simulink model "hx_model_alsop_20stages"  (R2017b)
settings: Solver=FixedStepAuto  StartTime=0.0  StopTime=Tsim  FixedStep=ST  RelTol=1e-3
values from neighbouring files (symbols this model uses):
  a1 = N_stages/(3600*Mc)    (= 0.000138888888889)    [main_open_loop_step_responses.m]    (also in main_pida_vs_pid_Fp_dist.m; main_pida_vs_pid_Tci_dist.m; main_pida_vs_pid_Tpi_dist.m; main_pida_vs_pid_sp.m)
  a2 = (U*A)/(3600*Mc*Cpc)    (= 0.010660331384)    [main_open_loop_step_responses.m]    (also in main_pida_vs_pid_Fp_dist.m; main_pida_vs_pid_Tci_dist.m; main_pida_vs_pid_Tpi_dist.m; main_pida_vs_pid_sp.m)
  a3 = N_stages/(3600*Mp)    (= 0.00037037037037)    [main_open_loop_step_responses.m]    (also in main_pida_vs_pid_Fp_dist.m; main_pida_vs_pid_Tci_dist.m; main_pida_vs_pid_Tpi_dist.m; main_pida_vs_pid_sp.m)
  a4 = (U*A)/(3600*Mp*Cpp)    (= 0.0341130604288)    [main_open_loop_step_responses.m]    (also in main_pida_vs_pid_Fp_dist.m; main_pida_vs_pid_Tci_dist.m; main_pida_vs_pid_Tpi_dist.m; main_pida_vs_pid_sp.m)
  Fc = 2500/7936.64    (= 0.314994758487)    [main_open_loop_step_responses.m]    (also in main_pida_vs_pid_Fp_dist.m; main_pida_vs_pid_Tci_dist.m; main_pida_vs_pid_Tpi_dist.m; main_pida_vs_pid_sp.m)
  Fp = 1500/7936.64    (= 0.188996855092)    [main_open_loop_step_responses.m]    (also in main_pida_vs_pid_Fp_dist.m; main_pida_vs_pid_Tci_dist.m; main_pida_vs_pid_Tpi_dist.m; main_pida_vs_pid_sp.m)
  step_Fc = -0.15    [main_open_loop_step_responses.m]    (also in main_tuning_pid.m = -0.05; main_tuning_pida.m = -0.05)
  step_time = 0    [main_open_loop_step_responses.m]    (also in main_pida_vs_pid_Fp_dist.m; main_pida_vs_pid_Tci_dist.m; main_pida_vs_pid_Tpi_dist.m; main_pida_vs_pid_sp.m)
  Tci = 294.26    [main_open_loop_step_responses.m]    (also in main_pida_vs_pid_Fp_dist.m; main_pida_vs_pid_Tci_dist.m; main_pida_vs_pid_Tpi_dist.m; main_pida_vs_pid_sp.m)
  Tco_init1 = Tco_init1.Data(end)    [main_open_loop_step_responses.m]    (also in main_pida_vs_pid_Fp_dist.m; main_pida_vs_pid_Tci_dist.m; main_pida_vs_pid_Tpi_dist.m; main_pida_vs_pid_sp.m)
  Tco_init10 = Tco_init10.Data(end)    [main_open_loop_step_responses.m]    (also in main_pida_vs_pid_Fp_dist.m; main_pida_vs_pid_Tci_dist.m; main_pida_vs_pid_Tpi_dist.m; main_pida_vs_pid_sp.m)
  Tco_init11 = Tco_init11.Data(end)    [main_open_loop_step_responses.m]    (also in main_pida_vs_pid_Fp_dist.m; main_pida_vs_pid_Tci_dist.m; main_pida_vs_pid_Tpi_dist.m; main_pida_vs_pid_sp.m)
  Tco_init12 = Tco_init12.Data(end)    [main_open_loop_step_responses.m]    (also in main_pida_vs_pid_Fp_dist.m; main_pida_vs_pid_Tci_dist.m; main_pida_vs_pid_Tpi_dist.m; main_pida_vs_pid_sp.m)
  Tco_init13 = Tco_init13.Data(end)    [main_open_loop_step_responses.m]    (also in main_pida_vs_pid_Fp_dist.m; main_pida_vs_pid_Tci_dist.m; main_pida_vs_pid_Tpi_dist.m; main_pida_vs_pid_sp.m)
  Tco_init14 = Tco_init14.Data(end)    [main_open_loop_step_responses.m]    (also in main_pida_vs_pid_Fp_dist.m; main_pida_vs_pid_Tci_dist.m; main_pida_vs_pid_Tpi_dist.m; main_pida_vs_pid_sp.m)
  Tco_init15 = Tco_init15.Data(end)    [main_open_loop_step_responses.m]    (also in main_pida_vs_pid_Fp_dist.m; main_pida_vs_pid_Tci_dist.m; main_pida_vs_pid_Tpi_dist.m; main_pida_vs_pid_sp.m)
  Tco_init16 = Tco_init16.Data(end)    [main_open_loop_step_responses.m]    (also in main_pida_vs_pid_Fp_dist.m; main_pida_vs_pid_Tci_dist.m; main_pida_vs_pid_Tpi_dist.m; main_pida_vs_pid_sp.m)
  Tco_init17 = Tco_init17.Data(end)    [main_open_loop_step_responses.m]    (also in main_pida_vs_pid_Fp_dist.m; main_pida_vs_pid_Tci_dist.m; main_pida_vs_pid_Tpi_dist.m; main_pida_vs_pid_sp.m)
  Tco_init18 = Tco_init18.Data(end)    [main_open_loop_step_responses.m]    (also in main_pida_vs_pid_Fp_dist.m; main_pida_vs_pid_Tci_dist.m; main_pida_vs_pid_Tpi_dist.m; main_pida_vs_pid_sp.m)
  Tco_init19 = Tco_init19.Data(end)    [main_open_loop_step_responses.m]    (also in main_pida_vs_pid_Fp_dist.m; main_pida_vs_pid_Tci_dist.m; main_pida_vs_pid_Tpi_dist.m; main_pida_vs_pid_sp.m)
  Tco_init2 = Tco_init2.Data(end)    [main_open_loop_step_responses.m]    (also in main_pida_vs_pid_Fp_dist.m; main_pida_vs_pid_Tci_dist.m; main_pida_vs_pid_Tpi_dist.m; main_pida_vs_pid_sp.m)
  Tco_init20 = Tco_init20.Data(end)    [main_open_loop_step_responses.m]    (also in main_pida_vs_pid_Fp_dist.m; main_pida_vs_pid_Tci_dist.m; main_pida_vs_pid_Tpi_dist.m; main_pida_vs_pid_sp.m)
  Tco_init3 = Tco_init3.Data(end)    [main_open_loop_step_responses.m]    (also in main_pida_vs_pid_Fp_dist.m; main_pida_vs_pid_Tci_dist.m; main_pida_vs_pid_Tpi_dist.m; main_pida_vs_pid_sp.m)
  Tco_init4 = Tco_init4.Data(end)    [main_open_loop_step_responses.m]    (also in main_pida_vs_pid_Fp_dist.m; main_pida_vs_pid_Tci_dist.m; main_pida_vs_pid_Tpi_dist.m; main_pida_vs_pid_sp.m)
  Tco_init5 = Tco_init5.Data(end)    [main_open_loop_step_responses.m]    (also in main_pida_vs_pid_Fp_dist.m; main_pida_vs_pid_Tci_dist.m; main_pida_vs_pid_Tpi_dist.m; main_pida_vs_pid_sp.m)
  Tco_init6 = Tco_init6.Data(end)    [main_open_loop_step_responses.m]    (also in main_pida_vs_pid_Fp_dist.m; main_pida_vs_pid_Tci_dist.m; main_pida_vs_pid_Tpi_dist.m; main_pida_vs_pid_sp.m)
  Tco_init7 = Tco_init7.Data(end)    [main_open_loop_step_responses.m]    (also in main_pida_vs_pid_Fp_dist.m; main_pida_vs_pid_Tci_dist.m; main_pida_vs_pid_Tpi_dist.m; main_pida_vs_pid_sp.m)
  Tco_init8 = Tco_init8.Data(end)    [main_open_loop_step_responses.m]    (also in main_pida_vs_pid_Fp_dist.m; main_pida_vs_pid_Tci_dist.m; main_pida_vs_pid_Tpi_dist.m; main_pida_vs_pid_sp.m)
  Tco_init9 = Tco_init9.Data(end)    [main_open_loop_step_responses.m]    (also in main_pida_vs_pid_Fp_dist.m; main_pida_vs_pid_Tci_dist.m; main_pida_vs_pid_Tpi_dist.m; main_pida_vs_pid_sp.m)
  Tpi = 366.48    [main_open_loop_step_responses.m]    (also in main_pida_vs_pid_Fp_dist.m; main_pida_vs_pid_Tci_dist.m; main_pida_vs_pid_Tpi_dist.m; main_pida_vs_pid_sp.m)
  Tpo_init1 = Tpo_init1.Data(end)    [main_open_loop_step_responses.m]    (also in main_pida_vs_pid_Fp_dist.m; main_pida_vs_pid_Tci_dist.m; main_pida_vs_pid_Tpi_dist.m; main_pida_vs_pid_sp.m)
  Tpo_init10 = Tpo_init10.Data(end)    [main_open_loop_step_responses.m]    (also in main_pida_vs_pid_Fp_dist.m; main_pida_vs_pid_Tci_dist.m; main_pida_vs_pid_Tpi_dist.m; main_pida_vs_pid_sp.m)
  Tpo_init11 = Tpo_init11.Data(end)    [main_open_loop_step_responses.m]    (also in main_pida_vs_pid_Fp_dist.m; main_pida_vs_pid_Tci_dist.m; main_pida_vs_pid_Tpi_dist.m; main_pida_vs_pid_sp.m)
  Tpo_init12 = Tpo_init12.Data(end)    [main_open_loop_step_responses.m]    (also in main_pida_vs_pid_Fp_dist.m; main_pida_vs_pid_Tci_dist.m; main_pida_vs_pid_Tpi_dist.m; main_pida_vs_pid_sp.m)
  Tpo_init13 = Tpo_init13.Data(end)    [main_open_loop_step_responses.m]    (also in main_pida_vs_pid_Fp_dist.m; main_pida_vs_pid_Tci_dist.m; main_pida_vs_pid_Tpi_dist.m; main_pida_vs_pid_sp.m)
  Tpo_init14 = Tpo_init14.Data(end)    [main_open_loop_step_responses.m]    (also in main_pida_vs_pid_Fp_dist.m; main_pida_vs_pid_Tci_dist.m; main_pida_vs_pid_Tpi_dist.m; main_pida_vs_pid_sp.m)
  Tpo_init15 = Tpo_init15.Data(end)    [main_open_loop_step_responses.m]    (also in main_pida_vs_pid_Fp_dist.m; main_pida_vs_pid_Tci_dist.m; main_pida_vs_pid_Tpi_dist.m; main_pida_vs_pid_sp.m)
  Tpo_init16 = Tpo_init16.Data(end)    [main_open_loop_step_responses.m]    (also in main_pida_vs_pid_Fp_dist.m; main_pida_vs_pid_Tci_dist.m; main_pida_vs_pid_Tpi_dist.m; main_pida_vs_pid_sp.m)
  Tpo_init17 = Tpo_init17.Data(end)    [main_open_loop_step_responses.m]    (also in main_pida_vs_pid_Fp_dist.m; main_pida_vs_pid_Tci_dist.m; main_pida_vs_pid_Tpi_dist.m; main_pida_vs_pid_sp.m)
  Tpo_init18 = Tpo_init18.Data(end)    [main_open_loop_step_responses.m]    (also in main_pida_vs_pid_Fp_dist.m; main_pida_vs_pid_Tci_dist.m; main_pida_vs_pid_Tpi_dist.m; main_pida_vs_pid_sp.m)
  Tpo_init19 = Tpo_init19.Data(end)    [main_open_loop_step_responses.m]    (also in main_pida_vs_pid_Fp_dist.m; main_pida_vs_pid_Tci_dist.m; main_pida_vs_pid_Tpi_dist.m; main_pida_vs_pid_sp.m)
  Tpo_init2 = Tpo_init2.Data(end)    [main_open_loop_step_responses.m]    (also in main_pida_vs_pid_Fp_dist.m; main_pida_vs_pid_Tci_dist.m; main_pida_vs_pid_Tpi_dist.m; main_pida_vs_pid_sp.m)
  Tpo_init20 = Tpo_init20.Data(end)    [main_open_loop_step_responses.m]    (also in main_pida_vs_pid_Fp_dist.m; main_pida_vs_pid_Tci_dist.m; main_pida_vs_pid_Tpi_dist.m; main_pida_vs_pid_sp.m)
  Tpo_init3 = Tpo_init3.Data(end)    [main_open_loop_step_responses.m]    (also in main_pida_vs_pid_Fp_dist.m; main_pida_vs_pid_Tci_dist.m; main_pida_vs_pid_Tpi_dist.m; main_pida_vs_pid_sp.m)
  Tpo_init4 = Tpo_init4.Data(end)    [main_open_loop_step_responses.m]    (also in main_pida_vs_pid_Fp_dist.m; main_pida_vs_pid_Tci_dist.m; main_pida_vs_pid_Tpi_dist.m; main_pida_vs_pid_sp.m)
  Tpo_init5 = Tpo_init5.Data(end)    [main_open_loop_step_responses.m]    (also in main_pida_vs_pid_Fp_dist.m; main_pida_vs_pid_Tci_dist.m; main_pida_vs_pid_Tpi_dist.m; main_pida_vs_pid_sp.m)
  Tpo_init6 = Tpo_init6.Data(end)    [main_open_loop_step_responses.m]    (also in main_pida_vs_pid_Fp_dist.m; main_pida_vs_pid_Tci_dist.m; main_pida_vs_pid_Tpi_dist.m; main_pida_vs_pid_sp.m)
  Tpo_init7 = Tpo_init7.Data(end)    [main_open_loop_step_responses.m]    (also in main_pida_vs_pid_Fp_dist.m; main_pida_vs_pid_Tci_dist.m; main_pida_vs_pid_Tpi_dist.m; main_pida_vs_pid_sp.m)
  Tpo_init8 = Tpo_init8.Data(end)    [main_open_loop_step_responses.m]    (also in main_pida_vs_pid_Fp_dist.m; main_pida_vs_pid_Tci_dist.m; main_pida_vs_pid_Tpi_dist.m; main_pida_vs_pid_sp.m)
  Tpo_init9 = Tpo_init9.Data(end)    [main_open_loop_step_responses.m]    (also in main_pida_vs_pid_Fp_dist.m; main_pida_vs_pid_Tci_dist.m; main_pida_vs_pid_Tpi_dist.m; main_pida_vs_pid_sp.m)
(part 2 of 2)

== matlab function hx_model_alsop_20stages/Subsystem/MATLAB Function14 ==
  data: Tpi input; DeltaT_LM output; Tco input; Tpo input; Tci input
function DeltaT_LM = fcn(Tpi,Tco,Tpo,Tci)
    Delta_T1 = Tpi-Tco;
    Delta_T2 = Tpo-Tci;
    if Delta_T1~=Delta_T2
        DeltaT_LM = (Delta_T1-Delta_T2)/log(Delta_T1/Delta_T2);
    else
        DeltaT_LM = Delta_T1;
    end
end

== matlab function hx_model_alsop_20stages/Subsystem/MATLAB Function15 ==
  data: Tpi input; DeltaT_LM output; Tco input; Tpo input; Tci input
function DeltaT_LM = fcn(Tpi,Tco,Tpo,Tci)
    Delta_T1 = Tpi-Tco;
    Delta_T2 = Tpo-Tci;
    if Delta_T1~=Delta_T2
        DeltaT_LM = (Delta_T1-Delta_T2)/log(Delta_T1/Delta_T2);
    else
        DeltaT_LM = Delta_T1;
    end
end

== matlab function hx_model_alsop_20stages/Subsystem/MATLAB Function16 ==
  data: Tpi input; DeltaT_LM output; Tco input; Tpo input; Tci input
function DeltaT_LM = fcn(Tpi,Tco,Tpo,Tci)
    Delta_T1 = Tpi-Tco;
    Delta_T2 = Tpo-Tci;
    if Delta_T1~=Delta_T2
        DeltaT_LM = (Delta_T1-Delta_T2)/log(Delta_T1/Delta_T2);
    else
        DeltaT_LM = Delta_T1;
    end
end

== matlab function hx_model_alsop_20stages/Subsystem/MATLAB Function17 ==
  data: Tpi input; DeltaT_LM output; Tco input; Tpo input; Tci input
function DeltaT_LM = fcn(Tpi,Tco,Tpo,Tci)
    Delta_T1 = Tpi-Tco;
    Delta_T2 = Tpo-Tci;
    if Delta_T1~=Delta_T2
        DeltaT_LM = (Delta_T1-Delta_T2)/log(Delta_T1/Delta_T2);
    else
        DeltaT_LM = Delta_T1;
    end
end

== matlab function hx_model_alsop_20stages/Subsystem/MATLAB Function18 ==
  data: Tpi input; DeltaT_LM output; Tco input; Tpo input; Tci input
function DeltaT_LM = fcn(Tpi,Tco,Tpo,Tci)
    Delta_T1 = Tpi-Tco;
    Delta_T2 = Tpo-Tci;
    if Delta_T1~=Delta_T2
        DeltaT_LM = (Delta_T1-Delta_T2)/log(Delta_T1/Delta_T2);
    else
        DeltaT_LM = Delta_T1;
    end
end

== matlab function hx_model_alsop_20stages/Subsystem/MATLAB Function19 ==
  data: Tpi input; DeltaT_LM output; Tco input; Tpo input; Tci input
function DeltaT_LM = fcn(Tpi,Tco,Tpo,Tci)
    Delta_T1 = Tpi-Tco;
    Delta_T2 = Tpo-Tci;
    if Delta_T1~=Delta_T2
        DeltaT_LM = (Delta_T1-Delta_T2)/log(Delta_T1/Delta_T2);
    else
        DeltaT_LM = Delta_T1;
    end
end

== matlab function hx_model_alsop_20stages/Kelvin_to_Fahrenheit ==
  data: u input; y output
function y = fcn(u)

    y = (u-273.15)*(9/5)+32;
    
end

== matlab function hx_model_alsop_20stages/Kelvin_to_Fahrenheit1 ==
  data: u input; y output
function y = fcn(u)

    y = (u-273.15)*(9/5)+32;
    
end

== matlab function hx_model_alsop_20stages/Fahrenheit_to_Kelvin ==
  data: u input; y output
function y = fcn(u)

    y = (u - 32)*(5/9) + 273.15;
    
end

== matlab function hx_model_alsop_20stages/Fahrenheit_to_Kelvin1 ==
  data: u input; y output
function y = fcn(u)

    y = (u - 32)*(5/9) + 273.15;
    
end
